simulink model "MPC_example_2mass_2024a"  (R2024a)
settings: Solver=FixedStepAuto  StartTime=0.0  StopTime=t_sim  FixedStep=t_sample  RelTol=1e-3
values from neighbouring files (symbols this model uses):
  Ad = sys_d.a    [MPC_example.m]
  Bd = sys_d.b    [MPC_example.m]
  c1 = 3    [MPC_example.m]
  c2 = 2    [MPC_example.m]
  Cd = sys_d.c    [MPC_example.m]
  fr = -2*G'*Qs    [MPC_example.m]
  fu = -2*M'*Qurs*c    [MPC_example.m]
  fx = 2*G'*Qs*F    [MPC_example.m]
  H = 2 * (G'*Qs*G + Qus + M'*Qurs*M)    [MPC_example.m]
  k1 = 20    [MPC_example.m]
  k2 = 15    [MPC_example.m]
  m1 = 1    [MPC_example.m]
  m2 = 1.2    [MPC_example.m]
  Np = 10    [MPC_example.m]
  Q = 0.01*eye(m)    [MPC_example.m]
  R = 0.0001*eye(n)    [MPC_example.m]
  t_sample = 0.03    [MPC_example.m]
undefined symbols (not defined in the file or in its folder): m, n, p
libraries: simulink x2
settings Model: Creator=Yang  LastModifiedBy=tianyue

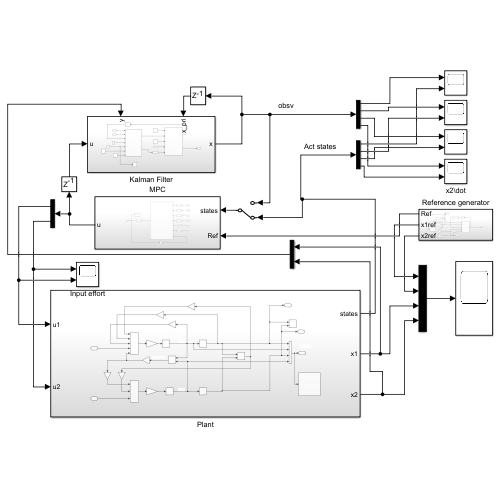
[thumbnail: Simulink's stored preview of the top-level diagram]
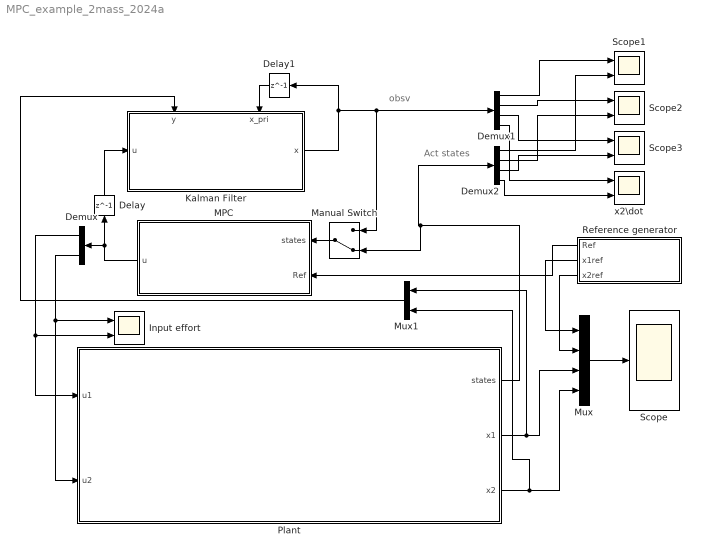
== system MPC_example_2mass_2024a ==
  note: Act states
  note: obsv
  Delay : Delay  DelayLength=1
  Delay1 : Delay  DelayLength=1
  Demux : Demux  Outputs=2
  Demux1 : Demux
  Demux2 : Demux
  Input effort : Scope  NumInputPorts=2
  Kalman Filter : Subsystem
      settings: PortSchema="{\"entries\":[{\"content\":{\"sides\":[{\"content\":{\"connectorIds\":[\"In1\"]},\"type\":\"ConnectorPlacement.EquallySpacedRectSide\",\"uuid\":\"8d922745-acf8-4b7c-9f7b-61e3c2970d4f\"},{\"content\":{\"connectorIds\":[\"Out1\"],\"side\":\"RIGHT\"},\"type\":\"ConnectorPlacement.EquallySpacedRectSide\",\"uuid\":\"dede757b-36c6-46c7-9196-56b7d8049f3e\"},{\"content\":{\"connectorIds\":[\"In2\",\"In3\"],\"side\":\"TOP\"},\"type\":\"ConnectorPlacement.EquallySpacedRectSide\",\"uuid\":\"ccf77bb7-b44e-4314-bebd-2ae52f6d6638\"}]},\"type\":\"ConnectorPlacement.EquallySpacedConnector\",\"uuid\":\"319e152c-4c54-4d1e-b875-a74a3bebb9b7\"}],\"packageUris\":[\"http://schema.mathworks.com/mf0/Connector/R2020b\"],\"version\":\"1.0\"}"
  MPC : Subsystem
  Manual Switch : ManualSwitch  CurrentSetting=0
  Mux : Mux
  Mux1 : Mux  Inputs=2
  Plant : Subsystem
  Reference generator : Subsystem
  Scope : Scope
  Scope1 : Scope  NumInputPorts=2
  Scope2 : Scope  NumInputPorts=2
  Scope3 : Scope  NumInputPorts=2
  x2\dot : Scope  NumInputPorts=2
  wires:
  Plant/1(states) -> Manual Switch/2, Demux2/1
  Reference generator/1(Ref) -> MPC/2(Ref)
  MPC/1(u) -> Demux/1, Delay/1
  Demux/1 -> Plant/1(u1), Input effort/2
  Demux/2 -> Input effort/1, Plant/2(u2)
  Mux/1 -> Scope/1
  Reference generator/2(x1ref) -> Mux/1
  Reference generator/3(x2ref) -> Mux/2
  Plant/2(x1) -> Mux1/1, Mux/3
  Plant/3(x2) -> Mux1/2, Mux/4
  Mux1/1 -> Kalman Filter/2(y)
  Delay/1 -> Kalman Filter/1(u)
  Kalman Filter/1(x) -> Demux1/1, Manual Switch/1, Delay1/1
  Delay1/1 -> Kalman Filter/3(x_pri)
  Demux1/1 -> Scope1/1
  Demux2/1 -> Scope1/2
  Demux1/2 -> Scope2/1
  Demux2/2 -> Scope2/2
  Demux1/3 -> Scope3/1
  Demux2/3 -> Scope3/2
  Demux1/4 -> x2\dot/1
  Demux2/4 -> x2\dot/2
  Manual Switch/1 -> MPC/1(states)

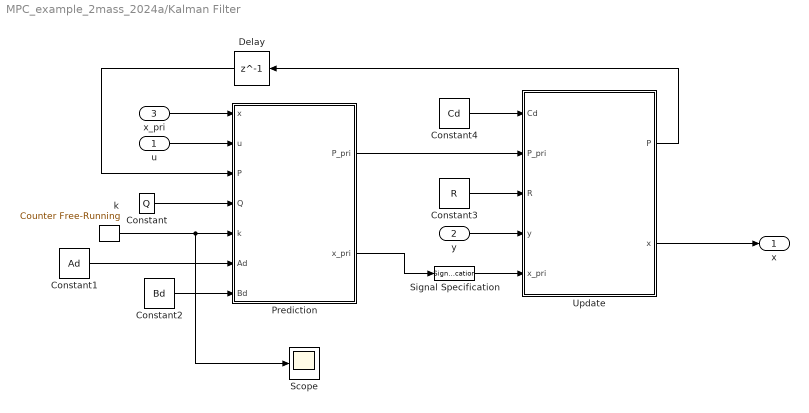
== system MPC_example_2mass_2024a/Kalman Filter ==
  u : Inport
  y : Inport  Port=2
  x_pri : Inport  Port=3
  Constant : Constant  Value=Q
  Constant1 : Constant  Value=Ad
  Constant2 : Constant  Value=Bd
  Constant3 : Constant  Value=R
  Constant4 : Constant  Value=Cd
  Delay : Delay  DelayLength=1  SampleTime=t_sample
  Prediction : MATLAB Function  TreatAsAtomicUnit=on
  Scope : Scope
  Signal Specification : SignalSpecification  Dimensions=[m,1]
  Update : MATLAB Function  TreatAsAtomicUnit=on
  k : simulink/Sources/Counter Free-Running  NumBits=16  tsamp=t_sample
  x : Outport
  wires:
  k/1 -> Scope/1, Prediction/5(k)
  u/1 -> Prediction/2(u)
  Constant/1 -> Prediction/4(Q)
  Constant1/1 -> Prediction/6(Ad)
  Constant2/1 -> Prediction/7(Bd)
  Prediction/1(P_pri) -> Update/2(P_pri)
  Prediction/2(x_pri) -> Signal Specification/1
  y/1 -> Update/4(y)
  Constant3/1 -> Update/3(R)
  Constant4/1 -> Update/1(Cd)
  Update/1(P) -> Delay/1
  Delay/1 -> Prediction/3(P)
  Update/2(x) -> x/1
  Signal Specification/1 -> Update/5(x_pri)
  x_pri/1 -> Prediction/1(x)

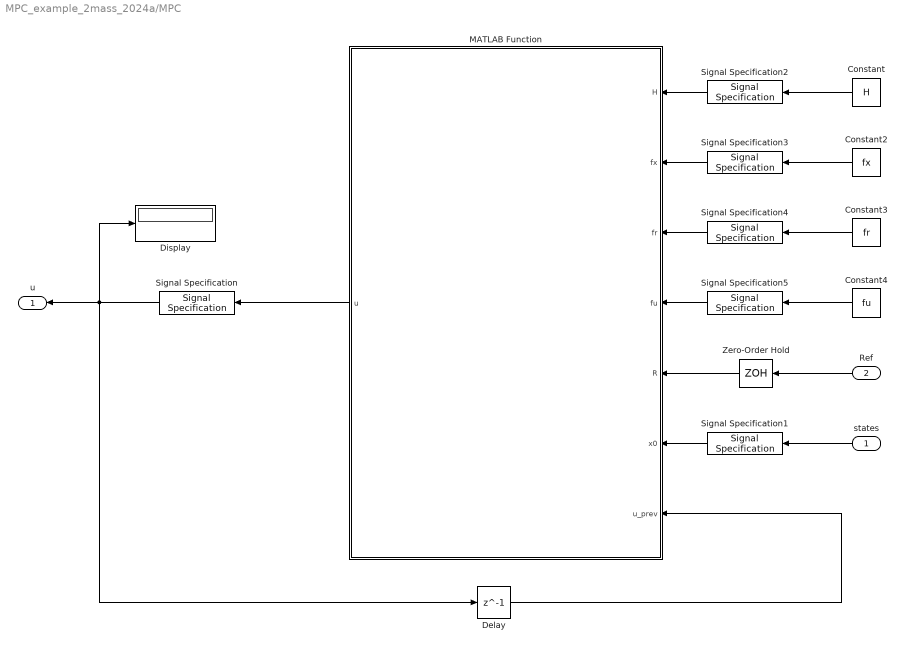
== system MPC_example_2mass_2024a/MPC ==
  states : Inport
  Ref : Inport  Port=2
  Constant : Constant  Value=H
  Constant2 : Constant  Value=fx
  Constant3 : Constant  Value=fr
  Constant4 : Constant  Value=fu
  Delay : Delay  DelayLength=1
  Display : Display
  MATLAB Function : MATLAB Function  TreatAsAtomicUnit=on
  Signal Specification : SignalSpecification  Dimensions=[p,1]
  Signal Specification1 : SignalSpecification  Dimensions=[m,1]
  Signal Specification2 : SignalSpecification  Dimensions=[Np*p,Np*p]
  Signal Specification3 : SignalSpecification  Dimensions=[p*Np,m]
  Signal Specification4 : SignalSpecification  Dimensions=[p*Np,n*Np]
  Signal Specification5 : SignalSpecification  Dimensions=[p*Np,p]
  Zero-Order Hold : ZeroOrderHold  SampleTime=t_sample
  u : Outport
  wires:
  Ref/1 -> Zero-Order Hold/1
  Zero-Order Hold/1 -> MATLAB Function/5(R)
  Constant/1 -> Signal Specification2/1
  states/1 -> Signal Specification1/1
  MATLAB Function/1(u) -> Signal Specification/1
  Signal Specification/1 -> Display/1, Delay/1, u/1
  Constant2/1 -> Signal Specification3/1
  Constant3/1 -> Signal Specification4/1
  Constant4/1 -> Signal Specification5/1
  Delay/1 -> MATLAB Function/7(u_prev)
  Signal Specification1/1 -> MATLAB Function/6(x0)
  Signal Specification2/1 -> MATLAB Function/1(H)
  Signal Specification3/1 -> MATLAB Function/2(fx)
  Signal Specification4/1 -> MATLAB Function/3(fr)
  Signal Specification5/1 -> MATLAB Function/4(fu)

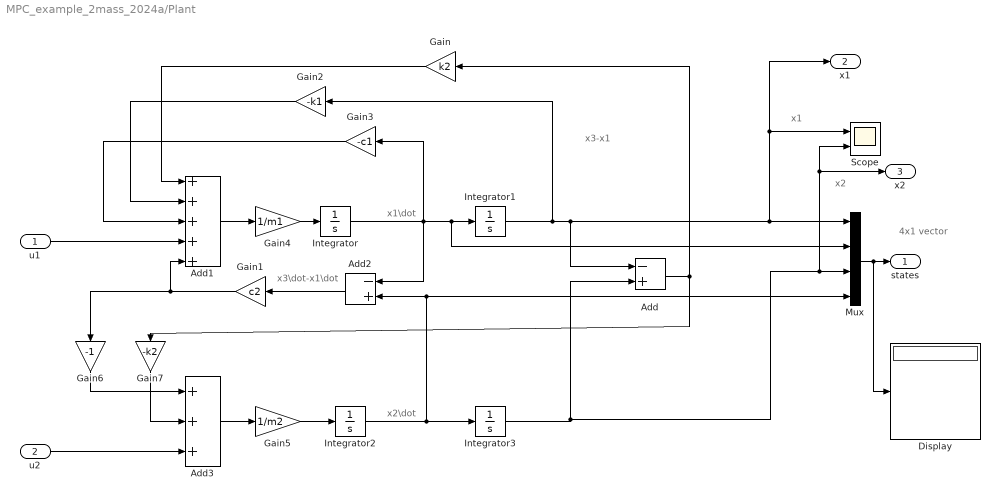
== system MPC_example_2mass_2024a/Plant ==
  note: 4x1 vector
  note: x2
  note: x1
  note: x3\dot-x1\dot
  note: x3-x1
  note: x2\dot
  note: x1\dot
  u1 : Inport
  u2 : Inport  Port=2
  Add : Sum  Inputs=-+
  Add1 : Sum  Inputs=+++++
  Add2 : Sum  Inputs=-+
  Add3 : Sum  Inputs=+++
  Display : Display
  Gain : Gain  Gain=k2
  Gain1 : Gain  Gain=c2
  Gain2 : Gain  Gain=-k1
  Gain3 : Gain  Gain=-c1
  Gain4 : Gain  Gain=1/m1
  Gain5 : Gain  Gain=1/m2
  Gain6 : Gain  Gain=-1
  Gain7 : Gain  Gain=-k2
  Integrator{,1..3} (4 alike) : Integrator
  Mux : Mux
  Scope : Scope  NumInputPorts=2
  states : Outport
  x1 : Outport  Port=2
  x2 : Outport  Port=3
  wires:
  Integrator/1 -> Gain3/1, Add2/1, Mux/2, Integrator1/1
  Integrator2/1 -> Mux/4, Add2/2, Integrator3/1
  Integrator1/1 -> Mux/1, x1/1, Scope/1, Add/1, Gain2/1
  Integrator3/1 -> x2/1, Scope/2, Mux/3, Add/2
  Add/1 -> Gain7/1, Gain/1
  Add1/1 -> Gain4/1
  u1/1 -> Add1/4
  Gain/1 -> Add1/1
  Add2/1 -> Gain1/1
  Gain1/1 -> Gain6/1, Add1/5
  Gain2/1 -> Add1/2
  Gain3/1 -> Add1/3
  Add3/1 -> Gain5/1
  u2/1 -> Add3/3
  Gain4/1 -> Integrator/1
  Gain5/1 -> Integrator2/1
  Gain6/1 -> Add3/1
  Gain7/1 -> Add3/2
  Mux/1 -> Display/1, states/1

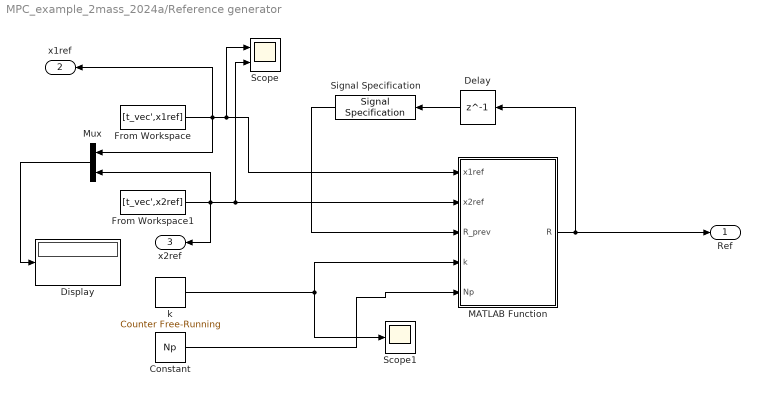
== system MPC_example_2mass_2024a/Reference generator ==
  Constant : Constant  Value=Np
  Delay : Delay  DelayLength=1  InitialCondition=0  SampleTime=t_sample
  Display : Display
  From Workspace : FromWorkspace  VariableName=[t_vec',x1ref]
  From Workspace1 : FromWorkspace  VariableName=[t_vec',x2ref]
  MATLAB Function : MATLAB Function  TreatAsAtomicUnit=on
  Mux : Mux  Inputs=2
  Scope : Scope  NumInputPorts=2
  Scope1 : Scope
  Signal Specification : SignalSpecification  Dimensions=[n*Np,1]
  k : simulink/Sources/Counter Free-Running  NumBits=16  tsamp=t_sample
  Ref : Outport
  x1ref : Outport  Port=2
  x2ref : Outport  Port=3
  wires:
  From Workspace1/1 -> x2ref/1, Mux/2, Scope/2, MATLAB Function/2(x2ref)
  From Workspace/1 -> x1ref/1, Mux/1, MATLAB Function/1(x1ref), Scope/1
  MATLAB Function/1(R) -> Ref/1, Delay/1
  Signal Specification/1 -> MATLAB Function/3(R_prev)
  k/1 -> MATLAB Function/4(k), Scope1/1
  Constant/1 -> MATLAB Function/5(Np)
  Delay/1 -> Signal Specification/1
  Mux/1 -> Display/1

== matlab function MPC_example_2mass_2024a/MPC/MATLAB Function ==
  data: H input; u output; fx input; fr input; fu input; R input; x0 input; u_prev input
function u = MPC(H,fx,fr,fu,R,x0,u_prev)
    
    p = 2;
    Np = 10;
    f = fx*x0 + fr*R + fu*u_prev;

    % Constrained MPC
    lb = -500*ones(p*Np,1);
    ub =  500*ones(p*Np,1);
    x0 = zeros(p*Np,1);
    options = optimoptions('quadprog','Algorithm','active-set');

    % U = -H\f;
    U = quadprog(H,f,[],[],[],[],lb,ub,x0,options);

    u = U(1:p);

    %u = u_prev + du;



end

== matlab function MPC_example_2mass_2024a/Reference generator/MATLAB Function ==
  data: x1ref input; x2ref input; R_prev input; R output; k input; Np input
function R = build_R_roll(x1ref,x2ref, R_prev, k, Np)
% ref    : n x 1 current reference
% R_prev : n*Np x 1 previous stacked reference
% k      : counter
% Np     : prediction horizon
ref = [x1ref;x2ref]; % 2x1
k = k+1;
n = 2; % number of outputs
Np = 10;

if k == 1
    R = repmat(ref, Np, 1);
else
    R = [R_prev(n+1:end); ref];
end

== matlab function MPC_example_2mass_2024a/Kalman Filter/Prediction ==
  data: P_pri output; x_pri output; x input; u input; P input; Q input; k input; Ad input; Bd input
function [P_pri,x_pri] = fcn(x,u,P,Q,k,Ad,Bd)


    % [m, ~] = size(Bd); % m states, p inputs
    m = 4;
    k = k+1;
    x0 = zeros(m,1); % initial states 
    P0 = 1*eye(m);
    


    if k == 1
        x = x0;
        x_pri = Ad*x + Bd*u; % update x pri   
        P = P0;
        P_pri = Ad*P*Ad' + Q; % Update Estimate cov pri

    else
        x_pri = Ad*x + Bd*u; % update x pri   
        P_pri = Ad*P*Ad' + Q; % Update Estimate cov pri
    end



end

== matlab function MPC_example_2mass_2024a/Kalman Filter/Update ==
  data: Cd input; P output; P_pri input; R input; y input; x output; x_pri input
function [P,x] = fcn(Cd,P_pri,R,y,x_pri)

    K = P_pri*Cd'*(Cd*P_pri*Cd' + R)^-1; % update Kalman gain


    x = x_pri + K*(y-Cd*x_pri); % state estimation 

    I = eye(size(K*Cd));
    P = (I-K*Cd)*P_pri;

end
